simulink library "NeuroMuscularLibrary"  (R2014b)
settings: Solver=ode45  StartTime=0.0  StopTime=10.0  RelTol=1e-3
values from neighbouring files (symbols this model uses):
  c = 0.05    [BodyMechParams.m]
  c_jointstop = 0.3 / (pi/180)    (= 17.1887338539)    [BodyMechParams.m]
  DeltaThRef = 2e-3    (= 0.002)    [BodyMechParams.m]
  eref = 0.04    [BodyMechParams.m]
  footBallToAnkleDist = 0.16    [BodyMechParams.m]
  footBallToCenterDist = footLength/2    (= 0.1)    [BodyMechParams.m]
  footBallToHeelDist = footLength    (= 0.2)    [BodyMechParams.m]
  footCenterToCGDist = 0.14 - footBallToCenterDist    (= 0.04)    [BodyMechParams.m]
  footInertia = 0.005    [BodyMechParams.m]
  footLength = 0.2    [BodyMechParams.m]
  footMass = 1.25    [BodyMechParams.m]
  g = 9.80665    [BodyMechParams.m]
  groundTheta = [atan(diff(groundZ)./diff(groundX)), 0]    [generateGround.m]
  groundZ = groundZ * stepSize/(largestStep+eps)    [generateGround.m]
  hatHipToCenterDistLen = hatLength/2    (= 0.4)    [BodyMechParams.m]
  hatInertia = 3    [BodyMechParams.m]
  hatLeftHipToCenterDistWidth = .15    (= 0.15)    [BodyMechParams.m]
  hatLength = 0.8    [BodyMechParams.m]
  hatMass = 53.5    [BodyMechParams.m]
  hatThickness = 0.2    [BodyMechParams.m]
  hatWidth = 0.4    [BodyMechParams.m]
  K = 5    [BodyMechParams.m]
  k_gn = k_gz    (= 78453.2)    [BodyMechParams.m]
  k_gt = k_gz    (= 78453.2)    [BodyMechParams.m]
  k_pressure = hatMass * g / DeltaThRef    (= 262327.8875)    [BodyMechParams.m]
  loptGAS = 0.05    [BodyMechParams.m]
  loptGLU = 0.11    [BodyMechParams.m]
  loptHAM = 0.10    (= 0.1)    [BodyMechParams.m]
  loptHFL = 0.11    [BodyMechParams.m]
  loptSOL = 0.04    [BodyMechParams.m]
  loptTA = 0.06    [BodyMechParams.m]
  loptVAS = 0.08    [BodyMechParams.m]
  lslackGAS = 0.40    (= 0.4)    [BodyMechParams.m]
  lslackGLU = 0.13    [BodyMechParams.m]
  lslackHAM = 0.31    [BodyMechParams.m]
  lslackHFL = 0.10    (= 0.1)    [BodyMechParams.m]
  lslackSOL = 0.26    [BodyMechParams.m]
  lslackTA = 0.24    [BodyMechParams.m]
  lslackVAS = 0.23    [BodyMechParams.m]
  mu_slide = 0.8    [BodyMechParams.m]
  mu_stick = 0.9    [BodyMechParams.m]
  N = 1.5    [BodyMechParams.m]    (also in cmaes.m = size(x,1))
  phimaxGASa = 20*pi/180    (= 0.349065850399)    [BodyMechParams.m]
  phimaxGASk = 40*pi/180    (= 0.698131700798)    [BodyMechParams.m]
  phimaxHAMk = 0*pi/180    (= 0)    [BodyMechParams.m]
  phimaxSOL = 20*pi/180    (= 0.349065850399)    [BodyMechParams.m]
  phimaxTA = -10*pi/180    (= -0.174532925199)    [BodyMechParams.m]
  phimaxVAS = 15*pi/180    (= 0.261799387799)    [BodyMechParams.m]
  phirefGASa = -10*pi/180    (= -0.174532925199)    [BodyMechParams.m]
  phirefGASk = 15*pi/180    (= 0.261799387799)    [BodyMechParams.m]
  phirefGLU = -30*pi/180    (= -0.523598775598)    [BodyMechParams.m]
  phirefHAMh = -25*pi/180    (= -0.436332312999)    [BodyMechParams.m]
  phirefHAMk = 0*pi/180    (= 0)    [BodyMechParams.m]
  phirefHFL = 0*pi/180    (= 0)    [BodyMechParams.m]
  phirefSOL = -10*pi/180    (= -0.174532925199)    [BodyMechParams.m]
  phirefTA = 20*pi/180    (= 0.349065850399)    [BodyMechParams.m]
  phirefVAS = 55*pi/180    (= 0.959931088597)    [BodyMechParams.m]
  rGASa = 0.05    [BodyMechParams.m]
  rGASk = 0.05    [BodyMechParams.m]
  rGLU = 0.10    (= 0.1)    [BodyMechParams.m]
  rHAMh = 0.08    [BodyMechParams.m]
  rHAMk = 0.05    [BodyMechParams.m]
  rHFL = 0.10    (= 0.1)    [BodyMechParams.m]
  rhoGASa = 0.7    [BodyMechParams.m]
  rhoGASk = 0.7    [BodyMechParams.m]
  rhoGLU = 0.5    [BodyMechParams.m]
  rhoHAMh = 0.7    [BodyMechParams.m]
  rhoHAMk = 0.7    [BodyMechParams.m]
  rhoHFL = 0.5    [BodyMechParams.m]
  rhoSOL = 0.5    [BodyMechParams.m]
  rhoTA = 0.7    [BodyMechParams.m]
  rhoVAS = 0.7    [BodyMechParams.m]
  rSOL = 0.05    [BodyMechParams.m]
  rTA = 0.04    [BodyMechParams.m]
  rVAS = 0.06    [BodyMechParams.m]
  s = x(1:N-1,:).^2 + x(2:N,:).^2    [cmaes.m]
  shankAnkleToCenterDist = shankLength/2    (= 0.25)    [BodyMechParams.m]
  shankAnkleToKneeDist = shankLength    (= 0.5)    [BodyMechParams.m]
  shankCenterToCGDist = 0.3 - shankAnkleToCenterDist    (= 0.05)    [BodyMechParams.m]
  shankInertia = 0.05    [BodyMechParams.m]
  shankLength = 0.5    [BodyMechParams.m]
  shankMass = 3.5    [BodyMechParams.m]
  tau = 0.01    [BodyMechParams.m]
  thighCenterToCGDist = 0.3 - thighKneeToCenterDist    (= 0.05)    [BodyMechParams.m]
  thighInertia = 0.15    [BodyMechParams.m]
  thighKneeToCenterDist = thighLength/2    (= 0.25)    [BodyMechParams.m]
  thighKneeToHipDist = thighLength    (= 0.5)    [BodyMechParams.m]
  thighLength = 0.5    [BodyMechParams.m]
  thighMass = 8.5    [BodyMechParams.m]
  v_gn_max = v_gz_max    (= 0.03)    [BodyMechParams.m]
  v_gt_max = v_gz_max    (= 0.03)    [BodyMechParams.m]
  v_max_pressure = 0.5    [BodyMechParams.m]
  vLimit = 0.01    [BodyMechParams.m]
  w = 0.56    [BodyMechParams.m]    (also in cmaes.m = ones(size(x,1)))
  w_max_jointstop = 1 * pi/180    (= 0.0174532925199)    [BodyMechParams.m]
undefined symbols (not defined in the file or in its folder): ankleBackDriveGain, ankleDgain, ankleFilterPID, ankleFilterSEA, ankleGearEff, ankleGearRatio, ankleIgain, ankleInitialAngle, ankleInputMass, ankleParallelSpringDamping, ankleParallelSpringOffset, ankleParallelSpringStiffness, anklePgain, ankleSEADamping, ankleSEAStiffness, ankleTendonMass, deltaLegAngleThr, footMassp, FourBarL1, FourBarL3, GainGAS, GainGLU, GainHAM, GainKneeOverExt, GainSOL, GainSOLTA, GainTA, GainVAS, hipDGain, hipPGain, Kglu, kneeAngleOffset, kneeBackDriveGain, kneeDgain, kneeExtendGain, kneeFilterPID, kneeFilterSEA, kneeFlexGain, kneeGearEff, kneeGearRatio, kneeHoldGain1, kneeHoldGain2, kneeIgain, kneeInitialAngle, kneePgain, kneeSEADamping, kneeSEAStiffness, kneeStatorMass, kneeStopGain, legAngleFilter, legAngleSpeedMax, legLengthClr, motorBackEMF, motorInductance, motorMaxCurrent, motorMaxVoltage, motorResistance, motorRotorInertia, motorRotorMass, motorTorsionalConst ... (+19)
undefined symbols (not defined in the file): ankleCJointstop, ankleIntCoulomb, ankleIntDamping, ankleIntStatic, anklePlantarLimit, ankleWMaxJointstop, dryFrictionDamping, dryFrictionStiffness, dryFrictionVelThresh, FmaxGLU, FT_GLU, kneeCJointstop, kneeExtCoulomb, kneeExtDamping, kneeExtStatic, kneeIntCoulomb, kneeIntDamping, kneeIntStatic, kneeWMaxJointstop, phiKneeUpLimit, RGainGAS, RGainGLU, RGainHAM, RGainHAMCut, RGainKneeOverExt, RGainSOL, RGainSOLTA, RGainTA, RGainVAS, RhipDGain, RhipPGain, RKglu, RkneeExtendGain, RkneeFlexGain, RkneeHoldGain1, RkneeHoldGain2, RkneeStopGain, RlegAngleFilter, RlegLengthClr, RPosGainGG, RSpeedGainGG
libraries: sm_lib x90, nesl_utility x44, simulink x18, dspswit3 x10, NeuroMuscularLibrary x8, simulink_extras x2
(part 1 of 5)
settings Model: Creator=nitisht  LastModifiedBy=Nitish

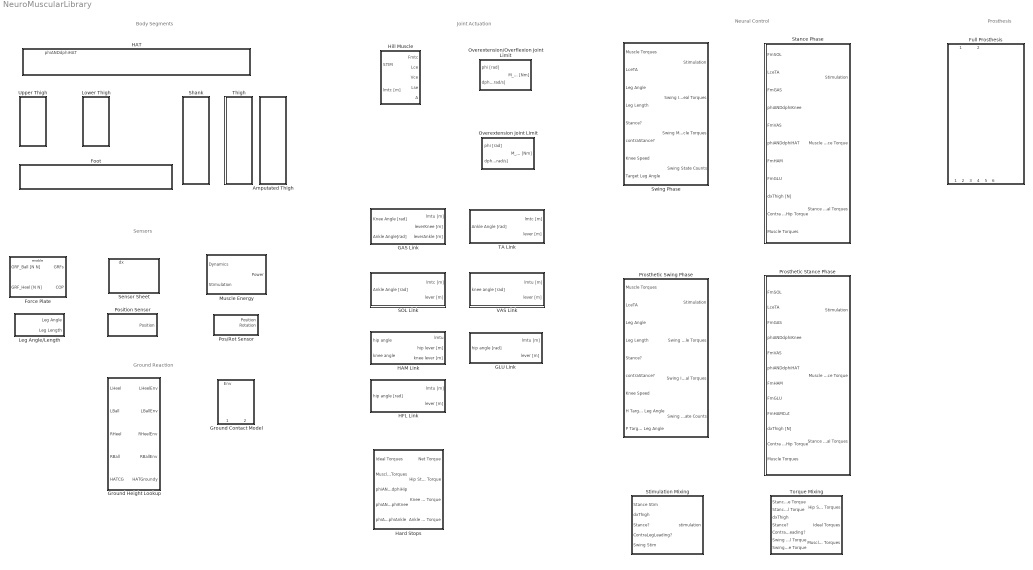
== system NeuroMuscularLibrary ==
  note: Body Segments
  note: Joint Actuation
  note: Sensors
  note: Ground Reaction
  note: Neural Control
  note: Prosthesis
  Amputated Thigh : Subsystem
  Foot : Subsystem
  Force Plate : Subsystem  TreatAsAtomicUnit=on
  Full Prosthesis : Subsystem
  GAS Link : Subsystem
  GLU Link : Subsystem
  Ground Contact Model : Subsystem
  Ground Height Lookup : Subsystem
  HAM Link : Subsystem
  HAT : Subsystem
  HFL Link : Subsystem
  Hard Stops : Subsystem
  Hill Muscle : Subsystem  mask(Hill Type Muscle){Fmax=0, lopt=0, vmax=0, lslack=0}
      mask prompts: Fmax "Max Isometric Force [N]"; lopt "Optimal Length [m]"; vmax "Max Contraction Velocity [m/s]"; lslack "Slack Length [m]"
      mask help:
      | Hill Type Muscle Model. This dialog allows you to specify several muscle-specific parameters. The block also requires several parameters to be defined globally in the matlab workspace:
      |
      | Excitation-contraction coupling parameters:
      | preA: preactivation
      | tau:  delay time constant [s]
      |
      | Contractile element (CE) force-length relationship:
      | w: width [lopt]
      | c: remaining force at +/- width
      |
      | CE force-velocity parameters:
      | N: eccentric force enhancement [Fmax]
      | K: shape factor
      |
      | Series elastic element (SE) force-length relationship
      | eref: tendon reference strain [lslack]
  Leg Angle/Length : Subsystem
  Lower Thigh : Subsystem
  Muscle Energy : Subsystem  mask{lopt=loptGLU, FT=FT_GLU, Fmax=FmaxGLU}
      mask prompts: lopt "Optimum Length:"; FT "Percent Fast Twitch"; Fmax "Max Iso Force"
  Overextension Joint Limit : Subsystem  mask{phiUpLimit=phiKneeUpLimit, ext=1}
      mask prompts: phiUpLimit "Upper Limit [rad]"; ext "Extension values are positive or negative?"
      mask help:
      | This block implements a hard joint limit that will prevent the joint from extending past the specified upper limit.
      |
      | Used for the knee and hip joints.
  Overextension/Overflexion Joint Limit : Subsystem  mask(Overextension/Overflexion Joint Limit){phiUpLimit=0, phiLowLimit=0}
      mask prompts: phiUpLimit "Upper Limit [rad]"; phiLowLimit "Lower Limit [rad]"
      mask help:
      | This block implents a hard joint limit that will prevent the joint from overextending past the specified upper limit and overflexing below the lower limit.
      |
      | Used for the Ankle Joint.
  Pos/Rot Sensor : Subsystem
  Position Sensor : Subsystem
  Prosthetic Stance Phase : Subsystem  mask{GainHAM=RGainHAM, GainHAMCut=RGainHAMCut, GainGLU=RGainGLU, GainSOL=RGainSOL, GainSOLTA=RGainSOLTA, GainTA=RGainTA, GainGAS=RGainGAS, GainVAS=RGainVAS, GainKneeOverExt=RGainKneeOverExt, PosGainGG=RPosGainGG, SpeedGainGG=RSpeedGainGG, Kglu=RKglu}
  Prosthetic Swing Phase : Subsystem  mask{GainTA=RGainTA, hipPGain=RhipPGain, hipDGain=RhipDGain, legAngleFilter=RlegAngleFilter, kneeFlexGain=RkneeFlexGain, kneeHoldGain1=RkneeHoldGain1, kneeHoldGain2=RkneeHoldGain2, kneeStopGain=RkneeStopGain, kneeExtendGain=RkneeExtendGain, legLengthClr=RlegLengthClr}
  SOL Link : Subsystem
  Sensor Sheet : Subsystem
  Shank : Subsystem
  Stance Phase : Subsystem  mask{GainHAM=GainHAM, GainGLU=GainGLU, GainSOL=GainSOL, GainSOLTA=GainSOLTA, GainTA=GainTA, GainGAS=GainGAS, GainVAS=GainVAS, GainKneeOverExt=GainKneeOverExt, PosGainGG=PosGainGG, SpeedGainGG=SpeedGainGG, Kglu=Kglu}
  Stimulation Mixing : Subsystem
  Swing Phase : Subsystem  mask{GainTA=GainTA, hipPGain=hipPGain, hipDGain=hipDGain, legAngleFilter=legAngleFilter, kneeFlexGain=kneeFlexGain, kneeHoldGain1=kneeHoldGain1, kneeHoldGain2=kneeHoldGain2, kneeStopGain=kneeStopGain, kneeExtendGain=kneeExtendGain, legLengthClr=legLengthClr}
  TA Link : Subsystem
  Thigh : Subsystem
  Torque Mixing : Subsystem
  Upper Thigh : Subsystem
  VAS Link : Subsystem

== system NeuroMuscularLibrary/Amputated Thigh ==
  Knee to Center : sm_lib/Frames and Transforms/Rigid Transform  TranslationMethod=Cartesian  TranslationLengthUnit=m  TranslationStandardAxis=+Z  TranslationStandardOffset=0  TranslationCartesianOffset=[0 thighKneeToCenterDist 0]  TranslationROffset=0  TranslationROffsetUnits=m  TranslationZOffset=0  TranslationZOffsetUnits=m  TranslationThetaOffset=0  TranslationThetaOffsetUnits=deg  RotationMethod=AlignedAxes  RotationAngleUnits=deg  RotationStandardAxis=+Z  RotationAngle=0  RotationArbitraryAxis=[0 0 1]  FollAlignAxisA=+Z  BaseAlignAxisA=+Y  FollAlignAxisB=+X  BaseAlignAxisB=+X  RotationMatrix=[1 0 0; 0 1 0; 0 0 1]  BlockFunction=simmechanics.library.frames_transforms.rigid_transform
  Knee to Center1 : sm_lib/Frames and Transforms/Rigid Transform  TranslationMethod=Cartesian  TranslationLengthUnit=m  TranslationStandardAxis=+Z  TranslationStandardOffset=0  TranslationCartesianOffset=[0 0 .05]  TranslationROffset=0  TranslationROffsetUnits=m  TranslationZOffset=0  TranslationZOffsetUnits=m  TranslationThetaOffset=0  TranslationThetaOffsetUnits=deg  RotationMethod=None  RotationAngleUnits=deg  RotationStandardAxis=+Z  RotationAngle=0  RotationArbitraryAxis=[0 0 1]  FollAlignAxisA=+Z  BaseAlignAxisA=+Y  FollAlignAxisB=+X  BaseAlignAxisB=+X  RotationMatrix=[1 0 0; 0 1 0; 0 0 1]  BlockFunction=simmechanics.library.frames_transforms.rigid_transform
  Knee to Sensor Sheet : sm_lib/Frames and Transforms/Rigid Transform  TranslationMethod=Cartesian  TranslationLengthUnit=m  TranslationStandardAxis=+Z  TranslationStandardOffset=0  TranslationCartesianOffset=[0 thighKneeToHipDist 0]  TranslationROffset=0  TranslationROffsetUnits=m  TranslationZOffset=0  TranslationZOffsetUnits=m  TranslationThetaOffset=0  TranslationThetaOffsetUnits=deg  RotationMethod=None  RotationAngleUnits=deg  RotationStandardAxis=+Z  RotationAngle=0  RotationArbitraryAxis=[0 0 1]  FollAlignAxisA=+Z  BaseAlignAxisA=+X  FollAlignAxisB=+Y  BaseAlignAxisB=+Y  RotationMatrix=[1 0 0; 0 1 0; 0 0 1]  BlockFunction=simmechanics.library.frames_transforms.rigid_transform
  Thigh CG : sm_lib/Frames and Transforms/Reference Frame  BlockFunction=simmechanics.library.frames_transforms.reference_frame
  Thigh Center to CG : sm_lib/Frames and Transforms/Rigid Transform  TranslationMethod=Cartesian  TranslationLengthUnit=m  TranslationStandardAxis=+Z  TranslationStandardOffset=0  TranslationCartesianOffset=[0 0 thighCenterToCGDist]  TranslationROffset=0  TranslationROffsetUnits=m  TranslationZOffset=0  TranslationZOffsetUnits=m  TranslationThetaOffset=0  TranslationThetaOffsetUnits=deg  RotationMethod=None  RotationAngleUnits=deg  RotationStandardAxis=+Z  RotationAngle=0  RotationArbitraryAxis=[0 0 1]  FollAlignAxisA=+X  BaseAlignAxisA=+Y  FollAlignAxisB=+Y  BaseAlignAxisB=+Z  RotationMatrix=[1 0 0; 0 1 0; 0 0 1]  BlockFunction=simmechanics.library.frames_transforms.rigid_transform
  Thigh Graphic : sm_lib/Body Elements/Solid  InertiaType=PointMass  Mass=0  MassUnits=kg  CenterOfMass=[0 0 thighCenterToCGDist]  CenterOfMassUnits=m  MomentsOfInertia=[thighInertia 0 0]  MomentsOfInertiaUnits=kg*m^2  ProductsOfInertia=[0 0 0]  ProductsOfInertiaUnits=kg*m^2  DensityBased=on  Density=1000  DensityUnits=kg/(m^3)  GraphicType=FromGeometry  MarkerShape=Sphere  MarkerSize=10  MarkerSizeUnits=m  GraphicVisPropType=SimpleVisualProperties  GraphicDiffuseColor=[0.5 0.5 0.5]  GraphicSpecularColor=[0.5 0.5 0.5 1.0]  GraphicAmbientColor=[0.15 0.15 0.15 1.0]  GraphicEmissiveColor=[0.0 0.0 0.0 1.0]  GraphicShininess=75  GraphicOpacity=1.0  GeometryShape=Cylinder  RectangleSize=[1 1]  RectangleSizeUnits=m  BrickDimensions=[1.05 .1]  BrickDimensionUnits=m  CylinderRadius=.075  CylinderRadiusUnits=m  CylinderLength=thighLength-.1  CylinderLengthUnits=m  SphereRadius=1  SphereRadiusUnits=m  EllipsoidRadii=[1 1 1]  EllipsoidRadiiUnits=m  ExtrusionCrossSection=[1 1; -1 1; -1 -1; 1 -1]  ExtrusionCrossSectionUnits=m  ExtrusionLength=1  ExtrusionLengthUnits=m  PolygonNumSides=3  PolygonOuterRadius=1  PolygonOuterRadiusUnits=m  ExtGeomFileType=STL  ExtGeomFileUnits=m  RevolutionCrossSection=[1 1; 1 -1; 2 -1; 2 1]  RevolutionCrossSectionUnits=m  RevolutionExtent=Full  RevolutionAngle=180  RevolutionAngleUnits=deg  BlockFunction=simmechanics.library.body_elements.solid
  Thigh inertia : sm_lib/Body Elements/Solid  InertiaType=Custom  Mass=thighMass  MassUnits=kg  CenterOfMass=[0 0 thighCenterToCGDist]  CenterOfMassUnits=m  MomentsOfInertia=[thighInertia 0 0]  MomentsOfInertiaUnits=kg*m^2  ProductsOfInertia=[0 0 0]  ProductsOfInertiaUnits=kg*m^2  DensityBased=on  Density=1000  DensityUnits=kg/(m^3)  GraphicType=None  MarkerShape=Sphere  MarkerSize=10  MarkerSizeUnits=m  GraphicVisPropType=SimpleVisualProperties  GraphicDiffuseColor=[0.5 0.5 0.5]  GraphicSpecularColor=[0.5 0.5 0.5 1.0]  GraphicAmbientColor=[0.15 0.15 0.15 1.0]  GraphicEmissiveColor=[0.0 0.0 0.0 1.0]  GraphicShininess=75  GraphicOpacity=1.0  GeometryShape=Cylinder  RectangleSize=[1 1]  RectangleSizeUnits=m  BrickDimensions=[1.05 .1]  BrickDimensionUnits=m  CylinderRadius=.075  CylinderRadiusUnits=m  CylinderLength=thighLength  CylinderLengthUnits=m  SphereRadius=1  SphereRadiusUnits=m  EllipsoidRadii=[1 1 1]  EllipsoidRadiiUnits=m  ExtrusionCrossSection=[1 1; -1 1; -1 -1; 1 -1]  ExtrusionCrossSectionUnits=m  ExtrusionLength=1  ExtrusionLengthUnits=m  PolygonNumSides=3  PolygonOuterRadius=1  PolygonOuterRadiusUnits=m  ExtGeomFileType=STL  ExtGeomFileUnits=m  RevolutionCrossSection=[1 1; 1 -1; 2 -1; 2 1]  RevolutionCrossSectionUnits=m  RevolutionExtent=Full  RevolutionAngle=180  RevolutionAngleUnits=deg  BlockFunction=simmechanics.library.body_elements.solid
  Knee : PMIOPort  Port=1  Side=Left
  Sensor Sheet : PMIOPort  Port=2  Side=Right
  connections:
  Knee/RConn1 -- Knee to Center/LConn1 -- Knee to Sensor Sheet/LConn1
  Knee to Center/RConn1 -- Knee to Center1/LConn1 -- Thigh inertia/RConn1 -- Thigh Center to CG/LConn1
  Knee to Sensor Sheet/RConn1 -- Sensor Sheet/RConn1
  Thigh Center to CG/RConn1 -- Thigh CG/RConn1
  Thigh Graphic/RConn1 -- Knee to Center1/RConn1

== system NeuroMuscularLibrary/Foot ==
  Ball To Ankle : sm_lib/Frames and Transforms/Rigid Transform  TranslationMethod=Cartesian  TranslationLengthUnit=m  TranslationStandardAxis=+Z  TranslationStandardOffset=0  TranslationCartesianOffset=[-footBallToAnkleDist 0 0]  TranslationROffset=0  TranslationROffsetUnits=m  TranslationZOffset=0  TranslationZOffsetUnits=m  TranslationThetaOffset=0  TranslationThetaOffsetUnits=deg  RotationMethod=None  RotationAngleUnits=deg  RotationStandardAxis=+Z  RotationAngle=0  RotationArbitraryAxis=[0 0 1]  FollAlignAxisA=+X  BaseAlignAxisA=+Y  FollAlignAxisB=+Y  BaseAlignAxisB=+Z  RotationMatrix=[1 0 0; 0 1 0; 0 0 1]  BlockFunction=simmechanics.library.frames_transforms.rigid_transform
  Ball To Heel : sm_lib/Frames and Transforms/Rigid Transform  TranslationMethod=Cartesian  TranslationLengthUnit=m  TranslationStandardAxis=+Z  TranslationStandardOffset=0  TranslationCartesianOffset=[-footBallToHeelDist 0 0]  TranslationROffset=0  TranslationROffsetUnits=m  TranslationZOffset=0  TranslationZOffsetUnits=m  TranslationThetaOffset=0  TranslationThetaOffsetUnits=deg  RotationMethod=None  RotationAngleUnits=deg  RotationStandardAxis=+Z  RotationAngle=0  RotationArbitraryAxis=[0 0 1]  FollAlignAxisA=+X  BaseAlignAxisA=+Y  FollAlignAxisB=+Y  BaseAlignAxisB=+Z  RotationMatrix=[1 0 0; 0 1 0; 0 0 1]  BlockFunction=simmechanics.library.frames_transforms.rigid_transform
  Ball to Center : sm_lib/Frames and Transforms/Rigid Transform  TranslationMethod=Cartesian  TranslationLengthUnit=m  TranslationStandardAxis=+Z  TranslationStandardOffset=0  TranslationCartesianOffset=[-footBallToCenterDist .025 0]  TranslationROffset=0  TranslationROffsetUnits=m  TranslationZOffset=0  TranslationZOffsetUnits=m  TranslationThetaOffset=0  TranslationThetaOffsetUnits=deg  RotationMethod=None  RotationAngleUnits=deg  RotationStandardAxis=+Z  RotationAngle=0  RotationArbitraryAxis=[0 0 1]  FollAlignAxisA=+X  BaseAlignAxisA=+Y  FollAlignAxisB=+Y  BaseAlignAxisB=+Z  RotationMatrix=[1 0 0; 0 1 0; 0 0 1]  BlockFunction=simmechanics.library.frames_transforms.rigid_transform
  Foot Solid : sm_lib/Body Elements/Solid  InertiaType=Custom  Mass=footMass  MassUnits=kg  CenterOfMass=[-footCenterToCGDist 0 0]  CenterOfMassUnits=m  MomentsOfInertia=[0 0 footInertia]  MomentsOfInertiaUnits=kg*m^2  ProductsOfInertia=[0 0 0]  ProductsOfInertiaUnits=kg*m^2  DensityBased=on  Density=1000  DensityUnits=kg/(m^3)  GraphicType=FromGeometry  MarkerShape=Sphere  MarkerSize=10  MarkerSizeUnits=m  GraphicVisPropType=SimpleVisualProperties  GraphicDiffuseColor=[0.5 0.5 0.5]  GraphicSpecularColor=[0.5 0.5 0.5 1.0]  GraphicAmbientColor=[0.15 0.15 0.15 1.0]  GraphicEmissiveColor=[0.0 0.0 0.0 1.0]  GraphicShininess=75  GraphicOpacity=1.0  GeometryShape=Brick  RectangleSize=[1 1]  RectangleSizeUnits=m  BrickDimensions=[footLength .05 .1]  BrickDimensionUnits=m  CylinderRadius=1  CylinderRadiusUnits=m  CylinderLength=1  CylinderLengthUnits=m  SphereRadius=1  SphereRadiusUnits=m  EllipsoidRadii=[1 1 1]  EllipsoidRadiiUnits=m  ExtrusionCrossSection=[1 1; -1 1; -1 -1; 1 -1]  ExtrusionCrossSectionUnits=m  ExtrusionLength=1  ExtrusionLengthUnits=m  PolygonNumSides=3  PolygonOuterRadius=1  PolygonOuterRadiusUnits=m  ExtGeomFileType=STL  ExtGeomFileUnits=m  RevolutionCrossSection=[1 1; 1 -1; 2 -1; 2 1]  RevolutionCrossSectionUnits=m  RevolutionExtent=Full  RevolutionAngle=180  RevolutionAngleUnits=deg  BlockFunction=simmechanics.library.body_elements.solid
  Ankle : PMIOPort  Port=1  Side=Right
  Heel : PMIOPort  Port=2  Side=Left
  Ball : PMIOPort  Port=3  Side=Left
  connections:
  Ball To Heel/LConn1 -- Ball to Center/LConn1 -- Ball/RConn1 -- Ball To Ankle/LConn1
  Ball to Center/RConn1 -- Foot Solid/RConn1
  Ball To Ankle/RConn1 -- Ankle/RConn1
  Ball To Heel/RConn1 -- Heel/RConn1

== system NeuroMuscularLibrary/Force Plate ==
  "GRF_Ball [N N] " : Inport
  GRF_Heel [N N] : Inport  Port=2
  Enable : EnablePort  StatesWhenEnabling=reset
  Fcn : Fcn  Expr=u(1)/(u(2)+eps)
  Mux : Mux  Inputs=3
  Mux1 : Mux  Inputs=2
  Selector : Selector  InputPortWidth=2  Indices=2
  Selector1 : Selector  InputPortWidth=2  Indices=2
  Sum1 : Sum
  GRFs : Outport  OutputWhenDisabled=reset  InitialOutput=0
  COP : Outport  Port=2  OutputWhenDisabled=reset  InitialOutput=0
  wires:
  Selector/1 -> Mux1/2
  Selector1/1 -> Mux1/1
  "GRF_Ball [N N] "/1 -> Sum1/1, Mux/1, Selector1/1
  GRF_Heel [N N]/1 -> Sum1/2, Mux/3
  Sum1/1 -> Mux/2, Selector/1
  Mux/1 -> GRFs/1
  Mux1/1 -> Fcn/1
  Fcn/1 -> COP/1

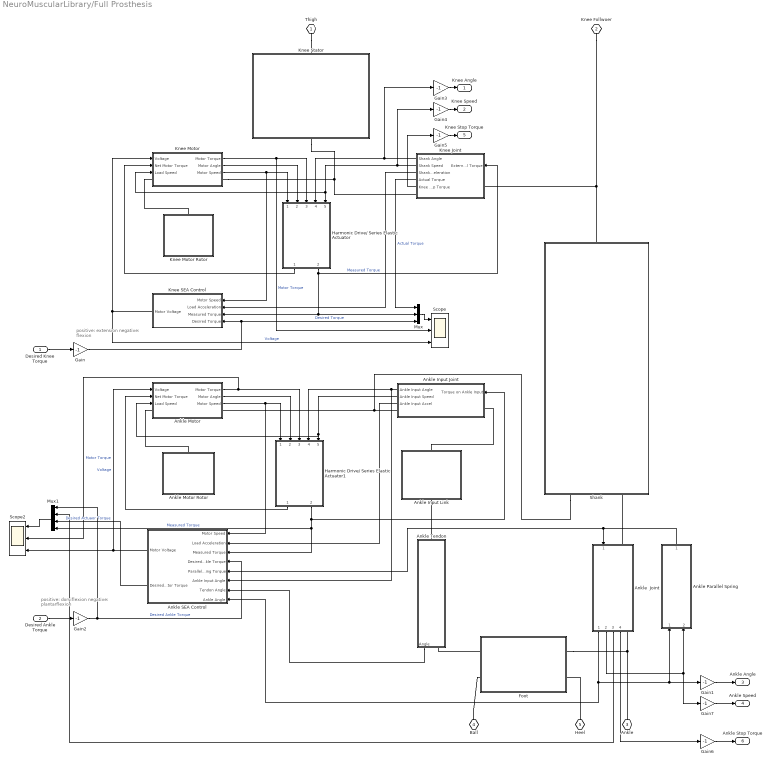
== system NeuroMuscularLibrary/Full Prosthesis ==
  note: positive: extension
      | negative: flexion
  note: positive: dorsiflexion
      | negative: plantarflexion
  Desired Knee Torque : Inport
  Desired Ankle Torque : Inport  Port=2
  Ankle  Joint : Subsystem
  Ankle Input Joint : Subsystem
  Ankle Input Link : Subsystem
      mask Display: image('ankleInputLinkThumb.png')
  Ankle Motor : Subsystem
  Ankle Motor Rotor : Subsystem
      mask Display: image('motorRotorThumb.png')
  Ankle Parallel Spring : Subsystem
  Ankle SEA Control : Subsystem
  Ankle Tendon : Subsystem
      mask Display: image('ankleTendonThumb.png')
  Foot : Subsystem
      mask Display: image('footThumb.png')
  Gain{,1..7} (8 alike) : Gain  Gain=-1
  Harmonic Drive/ Series Elastic Actuator : Subsystem
  Harmonic Drive/ Series Elastic Actuator1 : Subsystem
  Knee Joint : Subsystem
  Knee Motor : Subsystem
  Knee Motor Rotor : Subsystem
      mask Display: image('motorRotorThumb.png')
  Knee SEA Control : Subsystem
  Knee Stator : Subsystem
      mask Display: image('kneeStatorThumb.png')
  Mux : Mux  Inputs=3
  Mux1 : Mux
  Scope : Scope  NumInputPorts=3
      settings: ShowLegends=on  TimeRange=20  YMin=-100~-4.5~-50  YMax=50~4.5~50
  Scope2 : Scope  NumInputPorts=3
      settings: ShowLegends=on  TimeRange=1  YMin=-140~-4.5~-25  YMax=90~4.5~50
  Shank : Subsystem
      mask Display: image('shankThumb.png')
  Thigh : PMIOPort  Port=1  Side=Left
  Knee Follwoer : PMIOPort  Port=2  Side=Left
  Ankle : PMIOPort  Port=3  Side=Right
  Ball : PMIOPort  Port=4  Side=Right
  Heel : PMIOPort  Port=5  Side=Right
  Knee Angle : Outport
  Knee Speed : Outport  Port=2
  Ankle Angle : Outport  Port=3
  Ankle Speed : Outport  Port=4
  Knee Stop Torque : Outport  Port=5
  Ankle Stop Torque : Outport  Port=6
  wires:
  Ankle  Joint/4(Ankle Stop Torque) -> Gain6/1
  Gain6/1 -> Ankle Stop Torque/1
  Knee Joint/5(Knee Stop Torque) -> Gain5/1
  Gain5/1 -> Knee Stop Torque/1
  Ankle SEA Control/2(Desired Actuator Torque) -> Mux1/3  "Desired Actuaor Torque"
  Mux1/1 -> Scope2/1
  Gain2/1 -> Ankle SEA Control/4(Desired Ankle Torque), Mux1/1  "Desired Ankle Torque"
  Harmonic Drive/ Series Elastic Actuator1/2(Torque on Load) -> Ankle Input Joint/1(Torque on Ankle Input), Mux1/4, Ankle SEA Control/3(Measured Torque)  "Measured Torque"
  Ankle Motor/1(Motor Torque) -> Harmonic Drive/ Series Elastic Actuator1/3(Motor Torque), Scope2/2  "Motor Torque"
  Ankle SEA Control/1(Motor Voltage) -> Ankle Motor/1(Voltage), Scope2/3  "Voltage"
  Gain7/1 -> Ankle Speed/1
  Gain1/1 -> Ankle Angle/1
  Knee Joint/4(Actual Torque) -> Mux/1  "Actual Torque"
  Knee Motor/2(Motor Angle) -> Harmonic Drive/ Series Elastic Actuator/2(Motor Angle)
  Knee Motor/3(Motor Speed) -> Harmonic Drive/ Series Elastic Actuator/1(Motor Speed), Knee SEA Control/1(Motor Speed)
  Knee Motor/1(Motor Torque) -> Harmonic Drive/ Series Elastic Actuator/3(Motor Torque), Scope/2  "Motor Torque"
  Harmonic Drive/ Series Elastic Actuator/1(Torque on Motor) -> Knee Motor/2(Net Motor Torque)
  Knee Joint/1(Shank Angle) -> Gain3/1, Harmonic Drive/ Series Elastic Actuator/4(Load Angle)
  Knee Joint/2(Shank Speed) -> Gain4/1, Knee Motor/3(Load Speed), Harmonic Drive/ Series Elastic Actuator/5(Load Speed)
  Knee SEA Control/1(Motor Voltage) -> Scope/3, Knee Motor/1(Voltage)  "Voltage"
  Knee Joint/3(Shank Acceleration) -> Knee SEA Control/2(Load Acceleration)
  Ankle Motor/2(Motor Angle) -> Harmonic Drive/ Series Elastic Actuator1/2(Motor Angle)
  Ankle Motor/3(Motor Speed) -> Ankle SEA Control/1(Motor Speed), Harmonic Drive/ Series Elastic Actuator1/1(Motor Speed)
  Ankle Input Joint/1(Ankle Input Angle) -> Ankle SEA Control/6(Ankle Input Angle), Harmonic Drive/ Series Elastic Actuator1/4(Load Angle)
  Harmonic Drive/ Series Elastic Actuator1/1(Torque on Motor) -> Ankle Motor/2(Net Motor Torque)
  Ankle Input Joint/3(Ankle Input Accel) -> Ankle SEA Control/2(Load Acceleration)
  Ankle Tendon/1(Angle) -> Ankle SEA Control/7(Tendon Angle)
  Ankle Input Joint/2(Ankle Input Speed) -> Ankle Motor/3(Load Speed), Harmonic Drive/ Series Elastic Actuator1/5(Load Speed)
  Mux/1 -> Scope/1
  Gain/1 -> Mux/3, Knee SEA Control/4(Desired Torque)  "Desired Torque"
  Harmonic Drive/ Series Elastic Actuator/2(" Torque on Load") -> Knee SEA Control/3(Measured Torque), Mux/2, Knee Joint/1(External Torque)  "Measured Torque"
  Ankle Parallel Spring/1(Parallel Spring Torque) -> Ankle  Joint/1(Torque on Ankle), Ankle SEA Control/5(Parallel Spring Torque)
  Desired Knee Torque/1 -> Gain/1
  Desired Ankle Torque/1 -> Gain2/1
  Gain3/1 -> Knee Angle/1
  Gain4/1 -> Knee Speed/1
  Ankle  Joint/1(Ankle Angle) -> Ankle Parallel Spring/1(Ankle Angle), Gain1/1, Ankle SEA Control/8(Ankle Angle)
  Ankle  Joint/2(Ankle Speed) -> Ankle Parallel Spring/2(Ankle Speed), Gain7/1
  Ankle  Joint/3(Actual Torque) -> Mux1/2
  connections:
  Thigh/RConn1 -- Knee Stator/RConn1
  Knee Stator/LConn1 -- Knee Motor/RConn1 -- Knee Joint/RConn1
  Knee Motor Rotor/RConn1 -- Knee Motor/LConn1
  Shank/RConn1 -- Knee Joint/LConn1 -- Knee Follwoer/RConn1
  Shank/LConn1 -- Ankle Motor/RConn1 -- Ankle Input Joint/RConn1
  Ankle Motor Rotor/RConn1 -- Ankle Motor/LConn1
  Ankle Input Link/RConn1 -- Ankle Input Joint/LConn1
  Ankle  Joint/LConn1 -- Shank/LConn2
  Foot/RConn1 -- Ankle/RConn1 -- Ankle  Joint/RConn1
  Ankle Tendon/LConn1 -- Ankle Input Link/LConn1
  Foot/LConn1 -- Ankle Tendon/RConn1
  Ball/RConn1 -- Foot/LConn2
  Heel/RConn1 -- Foot/RConn2

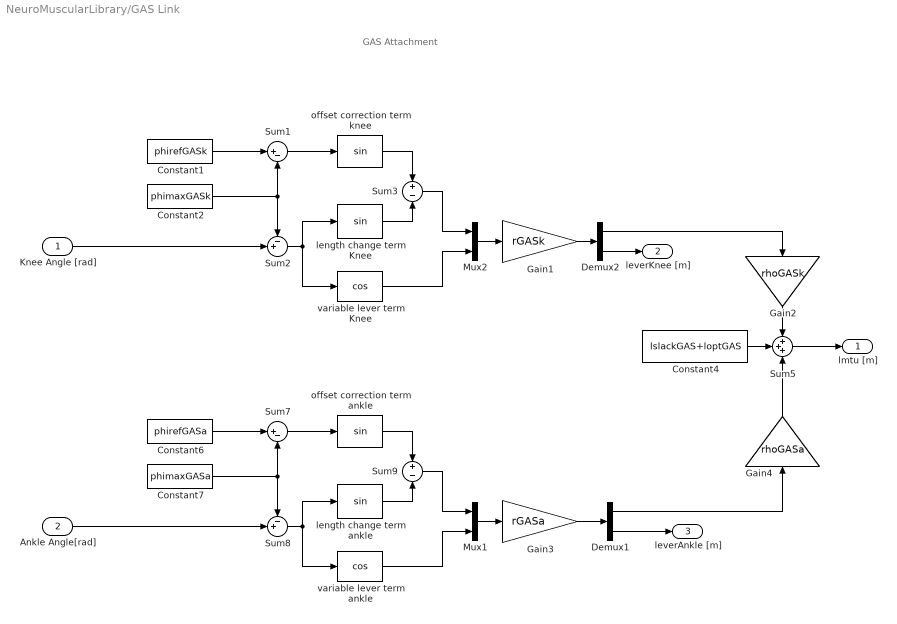
== system NeuroMuscularLibrary/GAS Link ==
  note: GAS Attachment
  Knee Angle [rad] : Inport
  Ankle Angle[rad] : Inport  Port=2
  Constant1 : Constant  Value=phirefGASk
  Constant2 : Constant  Value=phimaxGASk
  Constant4 : Constant  Value=lslackGAS+loptGAS
  Constant6 : Constant  Value=phirefGASa
  Constant7 : Constant  Value=phimaxGASa
  Demux1 : Demux  Outputs=2
  Demux2 : Demux  Outputs=2
  Gain1 : Gain  Gain=rGASk
  Gain2 : Gain  Gain=rhoGASk
  Gain3 : Gain  Gain=rGASa
  Gain4 : Gain  Gain=rhoGASa
  Mux1 : Mux  Inputs=2
  Mux2 : Mux  Inputs=2
  Sum1 : Sum  Inputs=|+-
  Sum2 : Sum  Inputs=-+|
  Sum3 : Sum  Inputs=+-
  Sum5 : Sum  Inputs=+++
  Sum7 : Sum  Inputs=|+-
  Sum8 : Sum  Inputs=-+|
  Sum9 : Sum  Inputs=+-
  length change term Knee : Trigonometry
  length change term ankle : Trigonometry
  offset correction term ankle : Trigonometry
  offset correction term knee : Trigonometry
  variable lever term Knee : Trigonometry  Operator=cos
  variable lever term ankle : Trigonometry  Operator=cos
  lmtu [m] : Outport
  leverKnee [m] : Outport  Port=2
  leverAnkle [m] : Outport  Port=3
  wires:
  Ankle Angle[rad]/1 -> Sum8/2
  Sum5/1 -> lmtu [m]/1
  variable lever term ankle/1 -> Mux1/2
  Demux1/2 -> leverAnkle [m]/1
  Sum8/1 -> variable lever term ankle/1, length change term ankle/1
  Constant7/1 -> Sum8/1, Sum7/2
  Sum7/1 -> offset correction term ankle/1
  Constant6/1 -> Sum7/1
  length change term ankle/1 -> Sum9/2
  offset correction term ankle/1 -> Sum9/1
  Sum9/1 -> Mux1/1
  Constant4/1 -> Sum5/2
  Mux1/1 -> Gain3/1
  Gain3/1 -> Demux1/1
  Demux1/1 -> Gain4/1
  Gain4/1 -> Sum5/3
  Knee Angle [rad]/1 -> Sum2/2
  variable lever term Knee/1 -> Mux2/2
  Sum2/1 -> variable lever term Knee/1, length change term Knee/1
  Constant2/1 -> Sum2/1, Sum1/2
  Sum1/1 -> offset correction term knee/1
  Constant1/1 -> Sum1/1
  length change term Knee/1 -> Sum3/2
  offset correction term knee/1 -> Sum3/1
  Sum3/1 -> Mux2/1
  Mux2/1 -> Gain1/1
  Gain1/1 -> Demux2/1
  Demux2/2 -> leverKnee [m]/1
  Demux2/1 -> Gain2/1
  Gain2/1 -> Sum5/1

== system NeuroMuscularLibrary/GLU Link ==
  note: GLUTEUS Attachment
  hip angle [rad] : Inport
  Constant : Constant  Value=lslackGLU+loptGLU
  Constant1 : Constant  Value=rGLU
  Constant2 : Constant  Value=phirefGLU
  Gain2 : Gain  Gain=rhoGLU
  Product : Product  RndMeth=Zero
  Sum2 : Sum  Inputs=|+-
  Sum5 : Sum  Inputs=|+-
  lmtu [m] : Outport
  lever [m] : Outport  Port=2
  wires:
  Constant/1 -> Sum5/1
  Sum5/1 -> lmtu [m]/1
  Product/1 -> Gain2/1
  hip angle [rad]/1 -> Sum2/1
  Constant2/1 -> Sum2/2
  Sum2/1 -> Product/1
  Constant1/1 -> Product/2, lever [m]/1
  Gain2/1 -> Sum5/2

== system NeuroMuscularLibrary/Ground Contact Model ==
  note: 2D Ground Interaction Model
  Env : Inport
  " contact sensor" : simulink/Logic and Bit Operations/Compare To Zero  relop=<=  OutDataTypeStr=boolean
  2D Contact : Subsystem
  Demux : Demux  Outputs=2
  Demux2 : Demux  Outputs=[1 2 2]
  External Force and Torque : sm_lib/Forces and Torques/External Force and Torque  ForceResolutionFrame=World  EnableForceX=on  EnableForceY=off  EnableForceZ=on  EnableForce=off  TorqueResolutionFrame=AttachedFrame  EnableTorqueX=off  EnableTorqueY=off  EnableTorqueZ=off  EnableTorque=off  BlockFunction=simmechanics.library.forces_torques.external_force_torque
  Mux1 : Mux  Inputs=2
  Mux2 : Mux  Inputs=2
  PS-Simulink Converter : nesl_utility/PS-Simulink Converter  PhysicalDomain=network_engine_domain  SubClassName=ps_output  LeftPortType=input  RightPortType=output  PseudoPeriodic=off  Frequencies=[]  Unit=m  AffineConversion=off
  PS-Simulink Converter1 : nesl_utility/PS-Simulink Converter  PhysicalDomain=network_engine_domain  SubClassName=ps_output  LeftPortType=input  RightPortType=output  PseudoPeriodic=off  Frequencies=[]  Unit=m/s  AffineConversion=off
  PS-Simulink Converter2 : nesl_utility/PS-Simulink Converter  PhysicalDomain=network_engine_domain  SubClassName=ps_output  LeftPortType=input  RightPortType=output  PseudoPeriodic=off  Frequencies=[]  Unit=m  AffineConversion=off
  PS-Simulink Converter3 : nesl_utility/PS-Simulink Converter  PhysicalDomain=network_engine_domain  SubClassName=ps_output  LeftPortType=input  RightPortType=output  PseudoPeriodic=off  Frequencies=[]  Unit=m/s  AffineConversion=off
  Simulink-PS Converter : nesl_utility/Simulink-PS Converter  PhysicalDomain=network_engine_domain  SubClassName=ps_input  LeftPortType=input  RightPortType=output  PseudoPeriodic=off  Frequencies=[]  NoiseDistribution=none  NoiseParameters=[]  Unit=1  AffineConversion=off  InputFiltering=off  SimscapeFilterOrder=1  InputFilterTimeConstant=0.001  UdotUserProvided=1
  Simulink-PS Converter1 : nesl_utility/Simulink-PS Converter  PhysicalDomain=network_engine_domain  SubClassName=ps_input  LeftPortType=input  RightPortType=output  PseudoPeriodic=off  Frequencies=[]  NoiseDistribution=none  NoiseParameters=[]  Unit=1  AffineConversion=off  InputFiltering=off  SimscapeFilterOrder=1  InputFilterTimeConstant=0.001  UdotUserProvided=1
  Sum : Sum  Inputs=-+|
  Sum1 : Sum
  Transform Sensor : sm_lib/Frames and Transforms/Transform Sensor  MeasurementFrame=World  SenseAngle=off  SenseAxis=off  SenseAngle1=off  SenseAngle2=off  SenseAngle3=off  SenseQ=off  SenseR=off  SenseOmegaX=off  SenseOmegaY=off  SenseOmegaZ=off  SenseOmega1=off  SenseOmega2=off  SenseOmega3=off  SenseQDot=off  SenseRDot=off  SenseAlphaX=off  SenseAlphaY=off  SenseAlphaZ=off  SenseAlpha1=off  SenseAlpha2=off  SenseAlpha3=off  SenseQDDot=off  SenseRDDot=off  SenseX=on  SenseY=off  SenseZ=on  SenseRad=off  SenseAzim=off  SenseDist=off  SenseInc=off  SenseXDot=on  SenseYDot=off  SenseZDot=on  SenseRadDot=off  SenseAzimDot=off  SenseDistDot=off  SenseIncDot=off  SenseXDDot=off  SenseYDDot=off  SenseZDDot=off  SenseRadDDot=off  SenseAzimDDot=off  SenseDistDDot=off  SenseIncDDot=off  BlockFunction=simmechanics.library.frames_transforms.transform_sensor
  World Frame : sm_lib/Frames and Transforms/World Frame  BlockFunction=simmechanics.library.frames_transforms.world_frame
  Foot : PMIOPort  Port=1  Side=Left
  Contact? : Outport
  GRF [N N] : Outport  Port=2
  wires:
  Demux/2 -> Simulink-PS Converter1/1
  Demux/1 -> Simulink-PS Converter/1
  Demux2/3 -> 2D Contact/2(nVec [m m])  "Normal Vector"
  Demux2/2 -> 2D Contact/1(RefPt [m m])  "Reference Point"
  Demux2/1 -> Sum/1  "Ground Height"
  Env/1 -> Demux2/1
  Mux2/1 -> 2D Contact/4(vVec [m/s m/s])
  2D Contact/2(FtVec [N N]) -> Sum1/2
  2D Contact/1(FnVec [N N]) -> Sum1/1
  Mux1/1 -> 2D Contact/3(pVec [m m])
  " contact sensor"/1 -> 2D Contact/Enable, Contact?/1
  PS-Simulink Converter1/1 -> Mux2/1
  PS-Simulink Converter/1 -> Mux1/1
  PS-Simulink Converter3/1 -> Mux2/2
  PS-Simulink Converter2/1 -> Sum/2, Mux1/2
  Sum/1 -> " contact sensor"/1
  Sum1/1 -> GRF [N N]/1, Demux/1
  connections:
  External Force and Torque/LConn1 -- Simulink-PS Converter/RConn1
  External Force and Torque/LConn2 -- Simulink-PS Converter1/RConn1
  Foot/RConn1 -- External Force and Torque/RConn1 -- Transform Sensor/RConn1
  Transform Sensor/LConn1 -- World Frame/RConn1
  Transform Sensor/RConn5 -- PS-Simulink Converter3/LConn1
  Transform Sensor/RConn4 -- PS-Simulink Converter1/LConn1
  Transform Sensor/RConn3 -- PS-Simulink Converter2/LConn1
  Transform Sensor/RConn2 -- PS-Simulink Converter/LConn1

== system NeuroMuscularLibrary/Ground Height Lookup ==
  LHeel : Inport
  LBall : Inport  Port=2
  RHeel : Inport  Port=3
  RBall : Inport  Port=4
  HATCG : Inport  Port=5
  Env Lookup : Subsystem
  Env Lookup1 : Subsystem
  Env Lookup2 : Subsystem
  Env Lookup3 : Subsystem
  Env Lookup4 : Subsystem
  Selector : Selector  InputPortWidth=5  Indices=[1]
  Selector{1..5} (5 alike) : Selector  InputPortWidth=3  Indices=[1]
  LHeelEnv : Outport  OutputWhenDisabled=reset  InitialOutput=0
  LBallEnv : Outport  Port=2  OutputWhenDisabled=reset  InitialOutput=0
  RHeelEnv : Outport  Port=3  OutputWhenDisabled=reset  InitialOutput=0
  RBallEnv : Outport  Port=4  OutputWhenDisabled=reset  InitialOutput=0
  HATGroundy : Outport  Port=5  OutputWhenDisabled=reset  InitialOutput=0
  wires:
  LHeel/1 -> Selector5/1
  LBall/1 -> Selector1/1
  RHeel/1 -> Selector3/1
  RBall/1 -> Selector4/1
  Selector5/1 -> Env Lookup/1(x)
  Env Lookup/1(Env) -> LHeelEnv/1
  Selector1/1 -> Env Lookup1/1(x)
  Env Lookup1/1(Env) -> LBallEnv/1
  Selector3/1 -> Env Lookup2/1(x)
  Selector4/1 -> Env Lookup3/1(x)
  Env Lookup2/1(Env) -> RHeelEnv/1
  Env Lookup3/1(Env) -> RBallEnv/1
  HATCG/1 -> Selector2/1
  Selector2/1 -> Env Lookup4/1(x)
  Env Lookup4/1(Env) -> Selector/1
  Selector/1 -> HATGroundy/1

== system NeuroMuscularLibrary/HAM Link ==
  note: HAM Attachment
  hip angle : Inport
  knee angle : Inport  Port=2
  Constant3 : Constant  Value=rHAMh
  Constant4 : Constant  Value=lslackHAM+loptHAM
  Constant5 : Constant  Value=phirefHAMh
  Constant6 : Constant  Value=phirefHAMk
  Constant7 : Constant  Value=phimaxHAMk  VectorParams1D=off
  Demux1 : Demux  Outputs=2
  Gain2 : Gain  Gain=rhoHAMh
  Gain3 : Gain  Gain=rHAMk
  Gain4 : Gain  Gain=rhoHAMk
  Mux1 : Mux  Inputs=2
  Product : Product  RndMeth=Zero
  Sum4 : Sum  Inputs=|+-
  Sum5 : Sum  Inputs=-++
  Sum7 : Sum  Inputs=|+-
  Sum8 : Sum  Inputs=-+|
  Sum9 : Sum  Inputs=+-
  length change term ankle : Trigonometry
  offset correction term ankle : Trigonometry
  variable lever term ankle : Trigonometry  Operator=cos
  lmtu : Outport
  hip lever [m] : Outport  Port=2
  knee lever [m] : Outport  Port=3
  wires:
  Constant5/1 -> Sum4/2
  Sum4/1 -> Product/1
  Constant3/1 -> hip lever [m]/1, Product/2
  Product/1 -> Gain2/1
  Sum5/1 -> lmtu/1
  variable lever term ankle/1 -> Mux1/2
  Demux1/2 -> knee lever [m]/1
  Sum8/1 -> variable lever term ankle/1, length change term ankle/1
  Constant7/1 -> Sum8/1, Sum7/2
  Sum7/1 -> offset correction term ankle/1
  Constant6/1 -> Sum7/1
  length change term ankle/1 -> Sum9/2
  offset correction term ankle/1 -> Sum9/1
  Sum9/1 -> Mux1/1
  Constant4/1 -> Sum5/2
  Mux1/1 -> Gain3/1
  Gain3/1 -> Demux1/1
  Demux1/1 -> Gain4/1
  Gain4/1 -> Sum5/3
  Gain2/1 -> Sum5/1
  hip angle/1 -> Sum4/1
  knee angle/1 -> Sum8/2

== system NeuroMuscularLibrary/HAT ==
  HAT CG : sm_lib/Frames and Transforms/Reference Frame  BlockFunction=simmechanics.library.frames_transforms.reference_frame
  HAT Center to CG : sm_lib/Frames and Transforms/Rigid Transform  TranslationMethod=Cartesian  TranslationLengthUnit=m  TranslationStandardAxis=+Z  TranslationStandardOffset=0  TranslationCartesianOffset=[0, 0, 0]  TranslationROffset=0  TranslationROffsetUnits=m  TranslationZOffset=0  TranslationZOffsetUnits=m  TranslationThetaOffset=0  TranslationThetaOffsetUnits=deg  RotationMethod=None  RotationAngleUnits=deg  RotationStandardAxis=+Z  RotationAngle=0  RotationArbitraryAxis=[0 0 1]  FollAlignAxisA=+X  BaseAlignAxisA=+Y  FollAlignAxisB=+Y  BaseAlignAxisB=+Z  RotationMatrix=[1 0 0; 0 1 0; 0 0 1]  BlockFunction=simmechanics.library.frames_transforms.rigid_transform
  HAT Center to Top : sm_lib/Frames and Transforms/Rigid Transform  TranslationMethod=StandardAxis  TranslationLengthUnit=m  TranslationStandardAxis=+Y  TranslationStandardOffset=hatLength/2  TranslationCartesianOffset=[0, 0, 0]  TranslationROffset=0  TranslationROffsetUnits=m  TranslationZOffset=0  TranslationZOffsetUnits=m  TranslationThetaOffset=0  TranslationThetaOffsetUnits=deg  RotationMethod=None  RotationAngleUnits=deg  RotationStandardAxis=+Z  RotationAngle=0  RotationArbitraryAxis=[0 0 1]  FollAlignAxisA=+X  BaseAlignAxisA=+Y  FollAlignAxisB=+Y  BaseAlignAxisB=+Z  RotationMatrix=[1 0 0; 0 1 0; 0 0 1]  BlockFunction=simmechanics.library.frames_transforms.rigid_transform
  Hip Solid : sm_lib/Body Elements/Solid  InertiaType=Custom  Mass=hatMass  MassUnits=kg  CenterOfMass=[0, 0, 0]  CenterOfMassUnits=m  MomentsOfInertia=[0 0 hatInertia]  MomentsOfInertiaUnits=kg*m^2  ProductsOfInertia=[0 0 0]  ProductsOfInertiaUnits=kg*m^2  DensityBased=on  Density=1000  DensityUnits=kg/(m^3)  GraphicType=FromGeometry  MarkerShape=Sphere  MarkerSize=10  MarkerSizeUnits=m  GraphicVisPropType=SimpleVisualProperties  GraphicDiffuseColor=[0.5 0.5 0.5]  GraphicSpecularColor=[0.5 0.5 0.5 1.0]  GraphicAmbientColor=[0.15 0.15 0.15 1.0]  GraphicEmissiveColor=[0.0 0.0 0.0 1.0]  GraphicShininess=75  GraphicOpacity=1.0  GeometryShape=Brick  RectangleSize=[1 1]  RectangleSizeUnits=m  BrickDimensions=[hatThickness, hatLength, hatWidth]  BrickDimensionUnits=m  CylinderRadius=1  CylinderRadiusUnits=m  CylinderLength=1  CylinderLengthUnits=m  SphereRadius=1  SphereRadiusUnits=m  EllipsoidRadii=[1 1 1]  EllipsoidRadiiUnits=m  ExtrusionCrossSection=[1 1; -1 1; -1 -1; 1 -1]  ExtrusionCrossSectionUnits=m  ExtrusionLength=1  ExtrusionLengthUnits=m  PolygonNumSides=3  PolygonOuterRadius=1  PolygonOuterRadiusUnits=m  ExtGeomFileType=STL  ExtGeomFileUnits=m  RevolutionCrossSection=[1 1; 1 -1; 2 -1; 2 1]  RevolutionCrossSectionUnits=m  RevolutionExtent=Full  RevolutionAngle=180  RevolutionAngleUnits=deg  BlockFunction=simmechanics.library.body_elements.solid
  Left Hip to Center : sm_lib/Frames and Transforms/Rigid Transform  TranslationMethod=Cartesian  TranslationLengthUnit=m  TranslationStandardAxis=+Z  TranslationStandardOffset=0  TranslationCartesianOffset=[0, hatHipToCenterDistLen, hatLeftHipToCenterDistWidth]  TranslationROffset=0  TranslationROffsetUnits=m  TranslationZOffset=0  TranslationZOffsetUnits=m  TranslationThetaOffset=0  TranslationThetaOffsetUnits=deg  RotationMethod=None  RotationAngleUnits=deg  RotationStandardAxis=+Z  RotationAngle=0  RotationArbitraryAxis=[0 0 1]  FollAlignAxisA=+X  BaseAlignAxisA=+Y  FollAlignAxisB=+Y  BaseAlignAxisB=+Z  RotationMatrix=[1 0 0; 0 1 0; 0 0 1]  BlockFunction=simmechanics.library.frames_transforms.rigid_transform
  Left Hip to Right Hip : sm_lib/Frames and Transforms/Rigid Transform  TranslationMethod=Cartesian  TranslationLengthUnit=m  TranslationStandardAxis=+Z  TranslationStandardOffset=0  TranslationCartesianOffset=[0 0 2*hatLeftHipToCenterDistWidth]  TranslationROffset=0  TranslationROffsetUnits=m  TranslationZOffset=0  TranslationZOffsetUnits=m  TranslationThetaOffset=0  TranslationThetaOffsetUnits=deg  RotationMethod=None  RotationAngleUnits=deg  RotationStandardAxis=+Z  RotationAngle=0  RotationArbitraryAxis=[0 0 1]  FollAlignAxisA=+X  BaseAlignAxisA=+Y  FollAlignAxisB=+Y  BaseAlignAxisB=+Z  RotationMatrix=[1 0 0; 0 1 0; 0 0 1]  BlockFunction=simmechanics.library.frames_transforms.rigid_transform
  Mux : Mux  Inputs=2
  PS-Simulink Converter : nesl_utility/PS-Simulink Converter  PhysicalDomain=network_engine_domain  SubClassName=ps_output  LeftPortType=input  RightPortType=output  PseudoPeriodic=off  Frequencies=[]  Unit=1  AffineConversion=off
  PS-Simulink Converter1 : nesl_utility/PS-Simulink Converter  PhysicalDomain=network_engine_domain  SubClassName=ps_output  LeftPortType=input  RightPortType=output  PseudoPeriodic=off  Frequencies=[]  Unit=1  AffineConversion=off
  To: X-forward Y-Lateral Z-up : sm_lib/Frames and Transforms/Rigid Transform  TranslationMethod=None  TranslationLengthUnit=m  TranslationStandardAxis=+Z  TranslationStandardOffset=0  TranslationCartesianOffset=[0, hatHipToCenterDistLen, -hatLeftHipToCenterDistWidth]  TranslationROffset=0  TranslationROffsetUnits=m  TranslationZOffset=0  TranslationZOffsetUnits=m  TranslationThetaOffset=0  TranslationThetaOffsetUnits=deg  RotationMethod=AlignedAxes  RotationAngleUnits=deg  RotationStandardAxis=+Z  RotationAngle=0  RotationArbitraryAxis=[0 0 1]  FollAlignAxisA=+X  BaseAlignAxisA=+X  FollAlignAxisB=+Z  BaseAlignAxisB=+Y  RotationMatrix=[1 0 0; 0 1 0; 0 0 1]  BlockFunction=simmechanics.library.frames_transforms.rigid_transform
  Transform Sensor : sm_lib/Frames and Transforms/Transform Sensor  MeasurementFrame=World  SenseAngle=on  SenseAxis=off  SenseAngle1=off  SenseAngle2=off  SenseAngle3=off  SenseQ=off  SenseR=off  SenseOmegaX=off  SenseOmegaY=on  SenseOmegaZ=off  SenseOmega1=off  SenseOmega2=off  SenseOmega3=off  SenseQDot=off  SenseRDot=off  SenseAlphaX=off  SenseAlphaY=off  SenseAlphaZ=off  SenseAlpha1=off  SenseAlpha2=off  SenseAlpha3=off  SenseQDDot=off  SenseRDDot=off  SenseX=off  SenseY=off  SenseZ=off  SenseRad=off  SenseAzim=off  SenseDist=off  SenseInc=off  SenseXDot=off  SenseYDot=off  SenseZDot=off  SenseRadDot=off  SenseAzimDot=off  SenseDistDot=off  SenseIncDot=off  SenseXDDot=off  SenseYDDot=off  SenseZDDot=off  SenseRadDDot=off  SenseAzimDDot=off  SenseDistDDot=off  SenseIncDDot=off  BlockFunction=simmechanics.library.frames_transforms.transform_sensor
  World Frame : sm_lib/Frames and Transforms/World Frame  BlockFunction=simmechanics.library.frames_transforms.world_frame
  Left Hip : PMIOPort  Port=1  Side=Left
  Right Hip : PMIOPort  Port=2  Side=Left
  HATTop : PMIOPort  Port=3  Side=Right
  CG : PMIOPort  Port=4  Side=Right
  phiANDdphiHAT : Outport
  wires:
  Mux/1 -> phiANDdphiHAT/1
  PS-Simulink Converter1/1 -> Mux/2
  PS-Simulink Converter/1 -> Mux/1
  connections:
  HATTop/RConn1 -- HAT Center to Top/RConn1
  CG/RConn1 -- HAT Center to CG/RConn1 -- HAT CG/RConn1
  To: X-forward Y-Lateral Z-up/RConn1 -- Transform Sensor/RConn1
  Transform Sensor/RConn3 -- PS-Simulink Converter1/LConn1
  PS-Simulink Converter/LConn1 -- Transform Sensor/RConn2
  Transform Sensor/LConn1 -- World Frame/RConn1
  Right Hip/RConn1 -- Left Hip to Right Hip/RConn1
  HAT Center to Top/LConn1 -- Hip Solid/RConn1 -- HAT Center to CG/LConn1 -- Left Hip to Center/RConn1
  Left Hip to Right Hip/LConn1 -- Left Hip to Center/LConn1 -- Left Hip/RConn1 -- To: X-forward Y-Lateral Z-up/LConn1

== system NeuroMuscularLibrary/HFL Link ==
  note: HFL Attachment
  hip angle [rad] : Inport
  Constant : Constant  Value=lslackHFL+loptHFL
  Constant1 : Constant  Value=rHFL
  Constant2 : Constant  Value=phirefHFL
  Gain2 : Gain  Gain=rhoHFL
  Product : Product  RndMeth=Zero
  Sum2 : Sum  Inputs=|+-
  Sum5 : Sum  Inputs=|++
  lmtu [m] : Outport
  lever [m] : Outport  Port=2
  wires:
  Constant/1 -> Sum5/1
  Sum5/1 -> lmtu [m]/1
  Product/1 -> Gain2/1
  hip angle [rad]/1 -> Sum2/1
  Constant2/1 -> Sum2/2
  Sum2/1 -> Product/1
  Constant1/1 -> Product/2, lever [m]/1
  Gain2/1 -> Sum5/2

== system NeuroMuscularLibrary/Hard Stops ==
  Ideal Torques : Inport
  Muscle Torques : Inport  Port=2
  phiANDdphiHip : Inport  Port=3
  phiANDdphiKnee : Inport  Port=4
  phiANDdphiAnkle : Inport  Port=5
  Add : Sum  Inputs=+++
  Ankle Joint Limit : NeuroMuscularLibrary/Overextension//Overflexion Joint Limit  phiUpLimit=phiAnkleUpLimit  phiLowLimit=phiAnkleLowLimit
  Demux : Demux  Outputs=2
  Demux1 : Demux  Outputs=2
  Demux2 : Demux  Outputs=2
  Hip Overextension Joint Limit : NeuroMuscularLibrary/Overextension Joint Limit  phiUpLimit=phiHipUpLimit  ext=1
  Knee Overextension Joint Limit : NeuroMuscularLibrary/Overextension Joint Limit  phiUpLimit=phiKneeUpLimit  ext=-1
  Mux : Mux  Inputs=3
  Over Extended Knee? : simulink/Logic and Bit Operations/Compare To Constant  relop=<  const=-5*pi/180  OutDataTypeStr=boolean
  Product1 : Product
  Net Torque : Outport
  Hip Stop Torque : Outport  Port=2
  Knee Stop Torque : Outport  Port=3
  Ankle Stop Torque : Outport  Port=4
  wires:
  Product1/1 -> Knee Stop Torque/1
  Knee Overextension Joint Limit/1 -> Mux/2, Product1/1
  Muscle Torques/1 -> Add/2
  Mux/1 -> Add/3
  Ankle Joint Limit/1 -> Ankle Stop Torque/1, Mux/3
  Over Extended Knee?/1 -> Product1/2
  Demux/2 -> Knee Overextension Joint Limit/2
  Demux/1 -> Over Extended Knee?/1, Knee Overextension Joint Limit/1
  Demux1/1 -> Hip Overextension Joint Limit/1
  Demux1/2 -> Hip Overextension Joint Limit/2
  Demux2/1 -> Ankle Joint Limit/1
  Demux2/2 -> Ankle Joint Limit/2
  phiANDdphiKnee/1 -> Demux/1
  Hip Overextension Joint Limit/1 -> Hip Stop Torque/1, Mux/1
  phiANDdphiHip/1 -> Demux1/1
  phiANDdphiAnkle/1 -> Demux2/1
  Add/1 -> Net Torque/1
  Ideal Torques/1 -> Add/1

== system NeuroMuscularLibrary/Hill Muscle ==
  note: Muscle-Tendon Dynamics
  note: Excitation Contraction Coupling
  STIM : Inport
  lmtc [m] : Inport  Port=2
  1 : Product  Inputs=**  SaturateOnIntegerOverflow=on  InputSameDT=on  OutDataTypeStr=Inherit: Same as first input
  1/lslack : Gain  Gain=1/lslack  SaturateOnIntegerOverflow=on  OutDataTypeStr=Inherit: Same as input  ParamDataTypeStr=Inherit: Same as input
  BE force-length relation : Subsystem
  CE force-length relation : Subsystem
  CE inverse force-velocity relation : Subsystem
  Constant : Constant  Value=lslack
  ECC TransferFcn : simulink_extras/Additional Linear/Transfer Fcn (with initial outputs)  N=[1]  D="[tau  1]"  Y0=preA  U0=0
      settings: AttributesFormatString=pre-activation: %<Y0>
  Fmax : Gain  Gain=Fmax  SaturateOnIntegerOverflow=on  OutDataTypeStr=Inherit: Same as input  ParamDataTypeStr=Inherit: Same as input
  Fv = Fse / (A*Fce) : Product  Inputs=*/  SaturateOnIntegerOverflow=on  InputSameDT=on  OutDataTypeStr=Inherit: Same as first input
  Integrator : Integrator  InitialConditionSource=external  LowerSaturationLimit=0.05
  PE force-length relation : Subsystem
  SE force-length relation : Subsystem
  Sum : Sum  Inputs=|+-  SaturateOnIntegerOverflow=on  InputSameDT=on  OutDataTypeStr=Inherit: Same as first input
  Sum2 : Sum  Inputs=|-+  SaturateOnIntegerOverflow=on  InputSameDT=on  OutDataTypeStr=Inherit: Same as first input
  Sum3 : Sum  SaturateOnIntegerOverflow=on  InputSameDT=on  OutDataTypeStr=Inherit: Same as first input
  Sum4 : Sum  SaturateOnIntegerOverflow=on  InputSameDT=on  OutDataTypeStr=Inherit: Same as first input
  lce/lopt : Gain  Gain=1/lopt  SaturateOnIntegerOverflow=on  OutDataTypeStr=Inherit: Same as input  ParamDataTypeStr=Inherit: Same as input
  vmax*lopt : Gain  Gain=vmax*lopt  SaturateOnIntegerOverflow=on  OutDataTypeStr=Inherit: Same as input  ParamDataTypeStr=Inherit: Same as input
  Fmtc : Outport  InitialOutput=0
  Lce : Outport  Port=2  InitialOutput=0
  Vce : Outport  Port=3  InitialOutput=0
  Lse : Outport  Port=4  InitialOutput=0
  A : Outport  Port=5  InitialOutput=0
  wires:
  Integrator/1 -> Sum/2, lce/lopt/1, Lce/1  "lce"
  Sum/1 -> 1/lslack/1, Lse/1  "lse"
  lce/lopt/1 -> CE force-length relation/1(lce [lopt]), BE force-length relation/1(lce [lopt]), PE force-length relation/1(lce [lopt])
  Fv = Fse / (A*Fce)/1 -> CE inverse force-velocity relation/1(Fv[Fmax])  "fv"
  vmax*lopt/1 -> Integrator/1, Vce/1  "vce"
  lmtc [m]/1 -> Sum2/2, Sum/1  "lmtc"
  Fmax/1 -> Fmtc/1  "Fmtc"
  1/lslack/1 -> SE force-length relation/1(lse [lslack])
  SE force-length relation/1(fse [Fmax]) -> Fmax/1, Sum4/1
  Sum2/1 -> Integrator/2
  Constant/1 -> Sum2/1
  CE force-length relation/1(fce [Fmax]) -> 1/1
  Sum4/1 -> Fv = Fse / (A*Fce)/1
  PE force-length relation/1(fpe [Fmax]) -> Sum3/1
  1/1 -> Sum3/2
  BE force-length relation/1(fbe [Fmax]) -> Sum4/2
  Sum3/1 -> Fv = Fse / (A*Fce)/2
  CE inverse force-velocity relation/1(v[vmax]) -> vmax*lopt/1
  STIM/1 -> ECC TransferFcn/1
  ECC TransferFcn/1 -> A/1, 1/2
